simulink model "Model_sfunc"  (R2023a)
settings: Solver=VariableStepAuto  StartTime=0.0  StopTime=20  RelTol=1e-3
InitFcn:
  | [modelDir, ~, ~] = fileparts(get_param(bdroot, 'FileName'));
  | run(fullfile(modelDir, 'startup_project.m'));
values from neighbouring files (symbols this model uses):
  p = struct()    [load_params.m]    (also in result_dir.m = fullfile(root, varargin{:}))
settings Model: Creator=Tan_Tram  LastModifiedBy=Tan_Tram

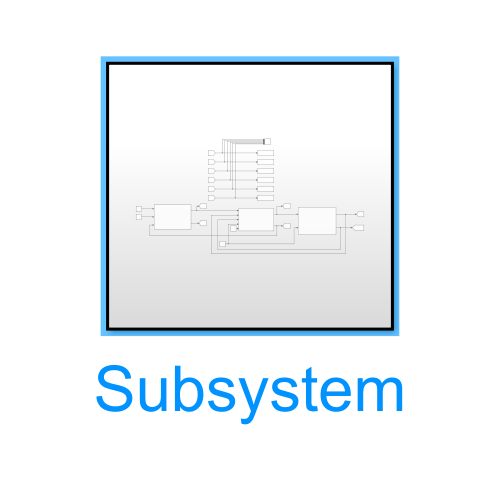
[thumbnail: Simulink's stored preview of the top-level diagram]
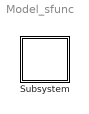
== system Model_sfunc ==
  Subsystem : Subsystem

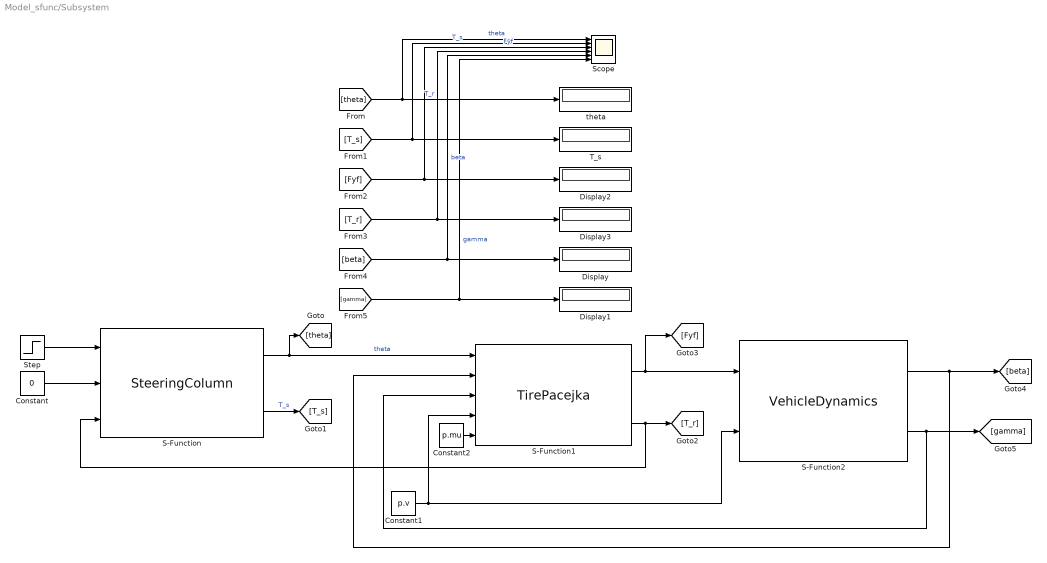
== system Model_sfunc/Subsystem ==
  Constant : Constant  Value=0
  Constant1 : Constant  Value=p.v
  Constant2 : Constant  Value=p.mu
  Display{,1..3} (4 alike) : Display
  S-Function : S-Function  FunctionName=SteeringColumn  Parameters=0.17198946,8.78410368,0.0052144  SFunctionDeploymentMode=off  EnableBusSupport=off  mask{J_total=p.J_total, B_total=p.B_total, T_f_total=p.T_f_total}
      mask prompts: J_total "J_total (kg·m^2)"; B_total "B_total (N·m/(rad/s))"; T_f_total "T_f_total (N·m)"
      mask Display:
      | disp('Steering Column');
      | 
      | port_label('input', 1, 'T_d');
      | port_label('input', 2, 'T_a');
      | port_label('input', 3, 'T_r');
      | port_label('output', 1, 'theta');
      | port_label('output', 2, 'T_s');
  S-Function1 : S-Function  FunctionName=TirePacejka  Parameters=0.0072,0.125,1.1,10,1.3,4500,-1,0.004032  SFunctionDeploymentMode=off  EnableBusSupport=off  mask{r_p=p.r_p, l_am=p.l_am, l_f=p.l_f, Bf=p.B, Cf=p.C, Df=p.D, Ef=p.E, K_torque_ratio=p.K_torque_ratio}
      mask prompts: r_p "r_p (m)"; l_am "l_am (m)"; l_f "l_f (m)"; Df "Df (N)"; K_torque_ratio "K_torque_ratio (m)"
      mask Display:
      | disp('Tire Pacejka');
      | 
      | port_label('input', 1, 'theta');
      | port_label('input', 2, 'beta');
      | port_label('input', 3, 'gamma');
      | port_label('input', 4, 'v');
      | port_label('input', 5, 'mu');
      | port_label('output', 1, 'Fyf');
      | port_label('output', 2, 'T_r');
  S-Function2 : S-Function  FunctionName=VehicleDynamics  Parameters=1573,1.1,1.58,50000,2873.16668925  SFunctionDeploymentMode=off  EnableBusSupport=off  mask{m=p.m, l_f=p.l_f, l_r=p.l_r, C_r=p.C_r, I_z=p.I_z}
      mask prompts: m "m (kg)"; l_f "l_f (m)"; l_r "l_r (m)"; C_r "C_r (N/rad)"; I_z "I_z (kg·m^2)"
      mask Display:
      | disp('Vehicle Dynamics');
      | 
      | port_label('input', 1, 'Fyf');
      | port_label('input', 2, 'v');
      | port_label('output', 1, 'beta');
      | port_label('output', 2, 'gamma');
  Scope : Scope  NumInputPorts=6
  Step : Step  Time=0  SampleTime=0
  T_s : Display
  theta : Display
  wires:
  S-Function2/2 -> [gamma], S-Function1/3
  S-Function/1 -> [theta], S-Function1/1  "theta"
  S-Function2/1 -> [beta], S-Function1/2
  S-Function1/1 -> S-Function2/1, [Fyf]
  Constant1/1 -> S-Function2/2, S-Function1/4
  Step/1 -> S-Function/1
  Constant/1 -> S-Function/2
  Constant2/1 -> S-Function1/5
  S-Function1/2 -> [T_r], S-Function/3
  S-Function/2 -> [T_s]  "T_s"
  [theta] -> Scope/1, theta/1  "theta"
  [T_s] -> Scope/2, T_s/1  "T_s"
  [Fyf] -> Scope/3, Display2/1  "Fyf"
  [gamma] -> Scope/6, Display1/1  "gamma"
  [beta] -> Scope/5, Display/1  "beta"
  [T_r] -> Scope/4, Display3/1  "T_r"
